simulink model "Final_Report_Simulink"  (R2016a)
settings: Solver=VariableStepAuto  StartTime=0.0  StopTime=4  RelTol=1e-3
settings Model: Creator=X1  LastModifiedBy=X1

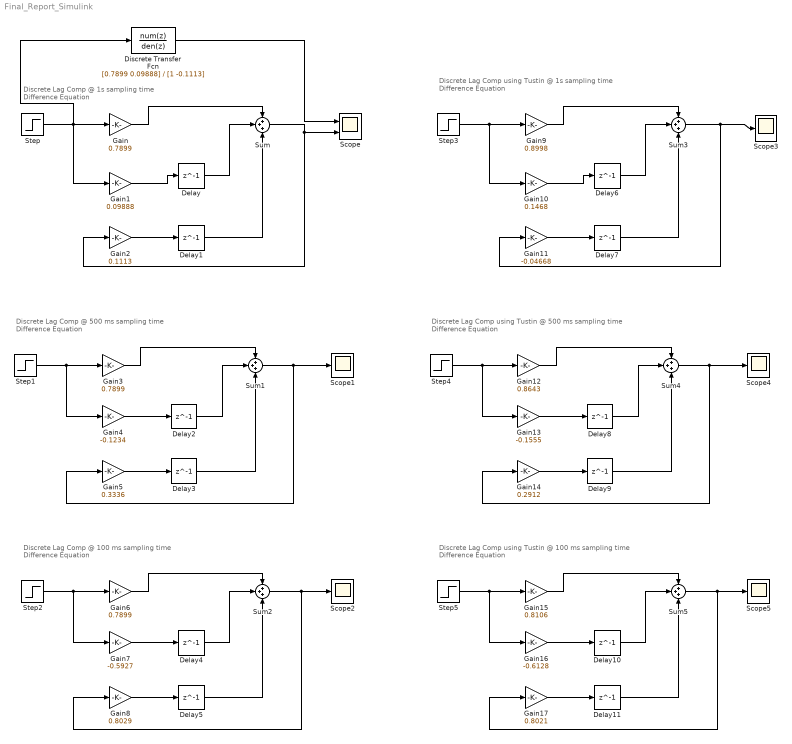
== system Final_Report_Simulink ==
  note: Discrete Lag Comp @ 1s sampling time
      | Difference Equation
  note: Discrete Lag Comp @ 500 ms sampling time
      | Difference Equation
  note: Discrete Lag Comp @ 100 ms sampling time
      | Difference Equation
  note: Discrete Lag Comp using Tustin @ 1s sampling time
      | Difference Equation
  note: Discrete Lag Comp using Tustin @ 500 ms sampling time
      | Difference Equation
  note: Discrete Lag Comp using Tustin @ 100 ms sampling time
      | Difference Equation
  Delay{,1,6..7} (4 alike) : Delay  DelayLength=1  InitialCondition=0  SampleTime=1
  Delay{4..5,10..11} (4 alike) : Delay  DelayLength=1  InitialCondition=0  SampleTime=0.1
  Delay{2..3,8..9} (4 alike) : Delay  DelayLength=1  InitialCondition=0  SampleTime=0.5
  Discrete Transfer Fcn : DiscreteTransferFcn  Numerator=[0.7899 0.09888]  Denominator=[1 -0.1113]  SampleTime=1
  Gain : Gain  Gain=0.7899
  Gain1 : Gain  Gain=0.09888
  Gain10 : Gain  Gain=0.1468
  Gain11 : Gain  Gain=-0.04668
  Gain12 : Gain  Gain=0.8643
  Gain13 : Gain  Gain=-0.1555
  Gain14 : Gain  Gain=0.2912
  Gain15 : Gain  Gain=0.8106
  Gain16 : Gain  Gain=-0.6128
  Gain17 : Gain  Gain=0.8021
  Gain2 : Gain  Gain=0.1113
  Gain3 : Gain  Gain=0.7899
  Gain4 : Gain  Gain=-0.1234
  Gain5 : Gain  Gain=0.3336
  Gain6 : Gain  Gain=0.7899
  Gain7 : Gain  Gain=-0.5927
  Gain8 : Gain  Gain=0.8029
  Gain9 : Gain  Gain=0.8998
  Scope : Scope  NumInputPorts=2
  Scope{1..5} (5 alike) : Scope
  Step : Step  SampleTime=1
  Step1 : Step  SampleTime=0.5
  Step2 : Step  SampleTime=0.1
  Step3 : Step  SampleTime=1
  Step4 : Step  SampleTime=0.5
  Step5 : Step  SampleTime=0.1
  Sum{,1..5} (6 alike) : Sum  Inputs=+++
  wires:
  Sum/1 -> Scope/2, Gain2/1
  Step/1 -> Discrete Transfer Fcn/1, Gain1/1, Gain/1
  Gain/1 -> Sum/1
  Gain2/1 -> Delay1/1
  Gain1/1 -> Delay/1
  Delay/1 -> Sum/2
  Delay1/1 -> Sum/3
  Sum1/1 -> Scope1/1, Gain5/1
  Step1/1 -> Gain4/1, Gain3/1
  Gain3/1 -> Sum1/1
  Gain5/1 -> Delay3/1
  Gain4/1 -> Delay2/1
  Delay2/1 -> Sum1/2
  Delay3/1 -> Sum1/3
  Sum2/1 -> Gain8/1, Scope2/1
  Step2/1 -> Gain7/1, Gain6/1
  Gain6/1 -> Sum2/1
  Gain8/1 -> Delay5/1
  Gain7/1 -> Delay4/1
  Delay4/1 -> Sum2/2
  Delay5/1 -> Sum2/3
  Sum3/1 -> Scope3/1, Gain11/1
  Step3/1 -> Gain10/1, Gain9/1
  Gain9/1 -> Sum3/1
  Gain11/1 -> Delay7/1
  Gain10/1 -> Delay6/1
  Delay6/1 -> Sum3/2
  Delay7/1 -> Sum3/3
  Sum4/1 -> Scope4/1, Gain14/1
  Step4/1 -> Gain13/1, Gain12/1
  Gain12/1 -> Sum4/1
  Gain14/1 -> Delay9/1
  Gain13/1 -> Delay8/1
  Delay8/1 -> Sum4/2
  Delay9/1 -> Sum4/3
  Sum5/1 -> Gain17/1, Scope5/1
  Step5/1 -> Gain16/1, Gain15/1
  Gain15/1 -> Sum5/1
  Gain17/1 -> Delay11/1
  Gain16/1 -> Delay10/1
  Delay10/1 -> Sum5/2
  Delay11/1 -> Sum5/3
  Discrete Transfer Fcn/1 -> Scope/1
